simulink model "tether_model_2"  (R2021b)
settings: Solver=VariableStepAuto  StartTime=0.0  StopTime=1.5*3600  RelTol=1e-3
model workspace (MAT data in the model file):
  At = 7.85398163397e-07
  Is = 1800595238.1
  L = 5000
  a = 7378
  ecc = 0.001
  gamma = 0.00015
  h_G = 1785.71428571
  m = 350
  me = 9.1093837e-31
  mu_m = 8.22e+22
  p = 0.0031
libraries: neural x139
(part 7 of 7)

== system tether_model_2/Feed-Forward Neural Network/Layer 5/Delays 1 ==
  "p{5}" : Inport  PortDimensions=32
      mask Display: e = 0.06;c1 = [120 230 180]/255;c2 = ([120 230 180]+0)/(256+128);c3 = ([120 230 180]+128)/(256+128);patch([0 1 1 0],[0 0 1 1],c1);patch([0 1 1 1-e 1-e 0+e],[0 0 1 1-e 0+e 0+e],c2);patch([0 0 1 1-e 0+e 0+e],[0 1 1 1-e 1-e 0+e],c3);plot([0 1 1 0 0],[0 0 1 1 0]);
  mux : Mux  Inputs=1
      mask Display: e = 0.06;c1 = [120 150 230]/255;c2 = ([120 150 230]+0)/383;c3 = ([120 150 230]+128)/383;patch([0 1 1 0],[0 0 1 1],c1);patch([0 1 1 1-e 1-e 0+e],[0 0 1 1-e 0+e 0+e],c2);patch([0 0 1 1-e 0+e 0+e],[0 1 1 1-e 1-e 0+e],c3);plot([0 1 1 0 0],[0 0 1 1 0]);disp('Mux')
  "pd{5,4}" : Outport
      mask Display: e = 0.06;c1 = [120 230 180]/255;c2 = ([120 230 180]+0)/(256+128);c3 = ([120 230 180]+128)/(256+128);patch([0 1 1 0],[0 0 1 1],c1);patch([0 1 1 1-e 1-e 0+e],[0 0 1 1-e 0+e 0+e],c2);patch([0 0 1 1-e 0+e 0+e],[0 1 1 1-e 1-e 0+e],c3);plot([0 1 1 0 0],[0 0 1 1 0]);
  wires:
  "p{5}"/1 -> mux/1
  mux/1 -> "pd{5,4}"/1

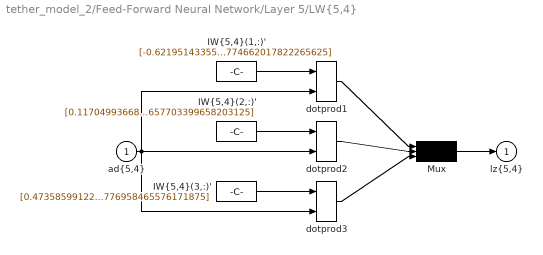
== system tether_model_2/Feed-Forward Neural Network/Layer 5/LW{5,4} ==
  "ad{5,4}" : Inport  PortDimensions=32
      mask Display: e = 0.06;c1 = [120 230 180]/255;c2 = ([120 230 180]+0)/(256+128);c3 = ([120 230 180]+128)/(256+128);patch([0 1 1 0],[0 0 1 1],c1);patch([0 1 1 1-e 1-e 0+e],[0 0 1 1-e 0+e 0+e],c2);patch([0 0 1 1-e 0+e 0+e],[0 1 1 1-e 1-e 0+e],c3);plot([0 1 1 0 0],[0 0 1 1 0]);
  "IW{5,4}(1,:)'" : Constant  Value=[-0.62195143355035809040742833531112410128116607666015625;0.204757317923436821249794093091622926294803619384765625;-0.300335195851072711548113147728145122528076171875;-0.07360812748318130982472240475544822402298450469970703125;-0.792060607860878729269415998714976012706756591796875;0.056090220190630375729501366777185467071831226348876953125;-0.460192982890725577060919704308616928756237030029296875;-0.2156401395735500770012293969557504169642925262451171875;0.3781651815348701095587102827266789972782135009765625;0.182449358825739038625357579803676344454288482666015625;-0.8124068724998851909191444065072573721408843994140625;0.99686560120035083709666423601447604596614837646484375;0.8548859964497144137141049213823862373828887939453125;0.471368357679506522206480667591677047312259674072265625;-0.74225418085054262196109675642219372093677520751953125;-0.50811740179140196804752349635236896574497222900390625;-0.08699430856769789499605138871629606001079082489013671875;0.17626293106978974112308833355200476944446563720703125;0.901505209672592844327709826757200062274932861328125;0.192819319263458577307090990871074609458446502685546875;-0.1488343844357109535536665134713985025882720947265625;-0.0743519786993882547676548711024224758148193359375;1.0321458358013513301187913384637795388698577880859375;0.1127084270811865296391118818064569495618343353271484375;-1.03056139100280663711828310624696314334869384765625;-0.81150148121102338993892999496893025934696197509765625;-0.11821508575096247029012630491706659086048603057861328125;0.08504380384017225236181758418751996941864490509033203125;0.75395417902985284452910264008096419274806976318359375;0.10092160925788225267485387348642689175903797149658203125;0.4384706426428817138685190002433955669403076171875;-0.45977774508780788753625756726250983774662017822265625]
      mask Display: e = 0.06;c1 = [120 150 230]/255;c2 = ([120 150 230]+0)/383;c3 = ([120 150 230]+128)/383;patch([0 1 1 0],[0 0 1 1],c1);patch([0 1 1 1-e 1-e 0+e],[0 0 1 1-e 0+e 0+e],c2);patch([0 0 1 1-e 0+e 0+e],[0 1 1 1-e 1-e 0+e],c3);plot([0 1 1 0 0],[0 0 1 1 0]);disp('weights');
  "IW{5,4}(2,:)'" : Constant  Value=[0.1170499366871233792863904454861767590045928955078125;-0.32708407884337187265799684610101394355297088623046875;0.478708075253142240068626733773271553218364715576171875;0.52559059568906330017767913886927999556064605712890625;0.260552228897964310849744151710183359682559967041015625;0.375021851984891851916614768924773670732975006103515625;-1.1164681773216489357736236343043856322765350341796875;0.464875249706074800126742729844409041106700897216796875;-0.360742076130005806522405009673093445599079132080078125;0.25025676258914331118177187818218953907489776611328125;0.367258700741840637959967352799139916896820068359375;-0.55567628299263327473767049013986252248287200927734375;-0.6277647777185795252563593749073334038257598876953125;-0.245924892057909294518225351566798053681850433349609375;-0.42742018018699734493992536954465322196483612060546875;0.38067959189806466202554702249472029507160186767578125;-0.2259224001307977569563689712595078162848949432373046875;-0.77198442013386381344020037431619130074977874755859375;-0.77707733974685233580004251052741892635822296142578125;0.19581128679648751589326138855540193617343902587890625;-0.45107343196972637944242023877450264990329742431640625;0.151971131808680548491707895664148963987827301025390625;0.084146090204320456162889740880928002297878265380859375;-0.1493240811492601294308002479738206602632999420166015625;-0.0304575164379494965627426239507258287630975246429443359375;-0.304097164877098091739782148579251952469348907470703125;-0.451200873198366714245111097625340335071086883544921875;0.85513455538690907875576385777094401419162750244140625;0.5945482263030330560837910525151528418064117431640625;0.48282330726073141580201308897812850773334503173828125;-0.244803318750227483224790603344445116817951202392578125;0.11076024144021918982350172200312954373657703399658203125]
      mask Display: e = 0.06;c1 = [120 150 230]/255;c2 = ([120 150 230]+0)/383;c3 = ([120 150 230]+128)/383;patch([0 1 1 0],[0 0 1 1],c1);patch([0 1 1 1-e 1-e 0+e],[0 0 1 1-e 0+e 0+e],c2);patch([0 0 1 1-e 0+e 0+e],[0 1 1 1-e 1-e 0+e],c3);plot([0 1 1 0 0],[0 0 1 1 0]);disp('weights');
  "IW{5,4}(3,:)'" : Constant  Value=[0.473585991225305813490109585472964681684970855712890625;0.6663465444866105702459435633500106632709503173828125;-0.2456992665310352708107899388778605498373508453369140625;0.378281168976102810663775244393036700785160064697265625;-0.1710741587325232127003715731916599906980991363525390625;-0.180429830712782568458152354651247151196002960205078125;-0.39599813397038918783010785773512907326221466064453125;0.289784496192740326225845137741998769342899322509765625;-0.66266444526163592598777540843002498149871826171875;0.716820604850110232320048453402705490589141845703125;-0.291571537794266755216909814407699741423130035400390625;-0.08258880437264130847108134503287146799266338348388671875;0.7348802772552149864537796020158566534519195556640625;0.729423167674049910402800378506071865558624267578125;0.50931861198151484604323968596872873604297637939453125;0.5327307495696016470532185849151574075222015380859375;0.62869955216386530505445762173621915280818939208984375;0.52236145441435455349932226454257033765316009521484375;0.9239413279772943354828385054133832454681396484375;0.394921144538807500357080471076187677681446075439453125;0.96086497796866876530685885882121510803699493408203125;0.59821828757363970652249918202869594097137451171875;0.1573707946132316681797647106577642261981964111328125;-0.219201608511633228015824670364963822066783905029296875;-0.500607302177475954607643870986066758632659912109375;0.76005796491962274163967094864347018301486968994140625;0.45021480723527229628189161303453147411346435546875;0.4763538541176599583337747390032745897769927978515625;-0.227899746591292140518447695285431109368801116943359375;0.75848112040483839368931739954859949648380279541015625;0.355304564601712835614222285585128702223300933837890625;0.4240867392359930487799601905862800776958465576171875]
      mask Display: e = 0.06;c1 = [120 150 230]/255;c2 = ([120 150 230]+0)/383;c3 = ([120 150 230]+128)/383;patch([0 1 1 0],[0 0 1 1],c1);patch([0 1 1 1-e 1-e 0+e],[0 0 1 1-e 0+e 0+e],c2);patch([0 0 1 1-e 0+e 0+e],[0 1 1 1-e 1-e 0+e],c3);plot([0 1 1 0 0],[0 0 1 1 0]);disp('weights');
  Mux : Mux  Inputs=3
      mask Display: e = 0.06;c1 = [120 150 230]/255;c2 = ([120 150 230]+0)/383;c3 = ([120 150 230]+128)/383;patch([0 1 1 0],[0 0 1 1],c1);patch([0 1 1 1-e 1-e 0+e],[0 0 1 1-e 0+e 0+e],c2);patch([0 0 1 1-e 0+e 0+e],[0 1 1 1-e 1-e 0+e],c3);plot([0 1 1 0 0],[0 0 1 1 0]);disp('Mux');
  dotprod1 : neural/Weight Functions/dotprod
  dotprod2 : neural/Weight Functions/dotprod
  dotprod3 : neural/Weight Functions/dotprod
  "lz{5,4}" : Outport
      mask Display: e = 0.06;c1 = [120 230 180]/255;c2 = ([120 230 180]+0)/(256+128);c3 = ([120 230 180]+128)/(256+128);patch([0 1 1 0],[0 0 1 1],c1);patch([0 1 1 1-e 1-e 0+e],[0 0 1 1-e 0+e 0+e],c2);patch([0 0 1 1-e 0+e 0+e],[0 1 1 1-e 1-e 0+e],c3);plot([0 1 1 0 0],[0 0 1 1 0]);
  wires:
  "IW{5,4}(1,:)'"/1 -> dotprod1/1
  "ad{5,4}"/1 -> dotprod1/2, dotprod2/2, dotprod3/2
  dotprod1/1 -> Mux/1
  "IW{5,4}(2,:)'"/1 -> dotprod2/1
  dotprod2/1 -> Mux/2
  "IW{5,4}(3,:)'"/1 -> dotprod3/1
  dotprod3/1 -> Mux/3
  Mux/1 -> "lz{5,4}"/1

== matlab function tether_model_2/MATLAB Function5 ==
  data: a input; Bx output; i input; ta input; mum input; By output; Bz output
function [Bx, By, Bz] = MagField(a, i, ta, mum)
    % Earthrs magnetic field vector in the Orbital Frame of SBET paper
    % SI units output

    % Define variables
    a = COES(1);
    i = COES(3);
    ta = COES(6);
    
%     Bo = 3.12e-5;
%     Bo_over_R3 = Bo/((p/(1+e*cos(ta)))/6378)^3;
    constant = mum/((a*1e3)^3);

    Bx = -2*constant*sin(i)*sin(ta);
    By = -constant*cos(i);
    Bz = constant*sin(i)*cos(ta);

== matlab function tether_model_2/MATLAB Function6 ==
  data: Bx input; a_r output; By input; Bz input; theta input; phi input; L input; Im input; m input; a_h output; a_theta output
function [a_r, a_h, a_theta] = edt_accelerations(Bx, By, Bz, theta, phi, L, Im, m)
    uhat = [cos(phi)*cos(theta), -sin(phi), cos(phi)*sin(theta)];
    f_orbital = Im*L*cross(uhat, [Bx, By, Bz]);
    a_orbital = f_orbital/m*1e-3'; % force to acceleraction in m to km
    a_r = a_orbital(1);
    a_h = a_orbital(2);
    a_theta = a_orbital(3);

== matlab function tether_model_2/MATLAB Function8 ==
  data: PHIe_0 input; h_0 input; Is input; ninf input; Em input; p input; At input; me input; e input; sigma input; mu input; gamma input; L input; Im output; fe output; mum input; mue_si input; h_G input
function [Im, fe] = find_current(PHIe_0, h_0, Is, ninf, Em, p, At, me, e, sigma, mu, gamma, L, mum, mue_si, h_G)
    h_span = [0, L];
    parameters = [p, At, me, Em, e, sigma, ninf, mu, gamma, h_0];
    opts = odeset( 'RelTol' , 1e-8 , 'AbsTol' , 1e-8 ) ;
    h = [];
    s = [];
    [h, s] = ode45( @current_distribution_diffe, h_span, [0, PHIe_0], opts, parameters) ;
    J1 = 0;
    Iint = 0;
    fe_right = 0;
    for ii = 2:length(h)
        J1 = J1 + ((h_G-h(ii))*(s(ii,1))+(h_G-h(ii-1))*(s(ii-1,1)))/2*(h(ii)-h(ii-1));
        Iint = Iint + (s(ii,1)+s(ii-1,1))/2*(h(ii)-h(ii-1));
        fe_right = fe_right + (h(ii)*s(ii,1) + h(ii-1)*s(ii-1,1))/2 * (h(ii)-h(ii-1));
    end
    epsilon = (J1/Is)*mum/mue_si;
    Im = Iint/L;
    fe = fe_right/(L^2*Im);

    function dstate = current_distribution_diffe(h,state,parameters) 
        Ie = real(state(1));
        PHIe = real(state(2));
    
        p = parameters(1); %perimeter in meters
        At = parameters(2);
        me = parameters(3); % mass of electron
        Em = parameters(4); % Induced electric field; dot(cross(v, B), u)
        e = parameters(5); % electron charge
        sigma = parameters(6); % from paper
        ninf = parameters(7); % ionospheric plasma density 
        mu = parameters(8); % apparently for atomic oxygen
        gamma = parameters(9);
        h0 = parameters(10);
    
        dstate = zeros(2,1);
        if real(h) < h0
            dstate(1) = e*ninf*p/pi*sqrt((2*e/me)*abs(PHIe));
        else
            dstate(1) = -e*ninf*p/pi*sqrt((2*e/me)*abs(PHIe))*mu*(1+gamma*abs(PHIe));
        end
        dstate(2) = Ie/(sigma*At)-Em;
    end
end

== matlab function tether_model_2/MATLAB Function9 ==
  data: output input; h_0 output; PHIe_0 output
function [h_0, PHIe_0] = fcn(output)

h_0 = output(1)*1e3;
PHIe_0 = output(3)*1e5;

== matlab function tether_model_2/MATLAB Function1 ==
  data: dtheta output; dphi output; Ttheta input; ddtheta output; Tphi input; Is input; theta input; phi input; dtheta input; dphi input; ddphi output
function [dtheta, dphi, ddtheta, ddphi] = fcn(Ttheta, Tphi, Is, theta, phi, dtheta, dphi)
    ddtheta = T(2)/Is;
    ddphi = T(3)/Is;

== matlab function tether_model_2/MATLAB Function ==
  data: mue input; a_r input; da output; a_h input; a_theta input; a input; ecc input; i input; RAAN input; aop input; ta input; decc output; di output; dRAAN output; daop output; dta output
function [da, decc, di, dRAAN, daop, dta]  = VoP(mue, a_r, a_h, a_theta, a, ecc, i, RAAN, aop, ta)
%     a = state(1);
%     ecc = state(2);
%     i = state(3);
%     RAAN = state(4);
%     aop = state(5);
%     ta = state(6);

    p = a*(1-ecc^2);
    h = sqrt(mue*p);
    r = p/(1+ecc*cos(ta));
    n = sqrt(mue/a^3);
    u = aop + ta;

    da = (2/(n*sqrt(1-ecc^2)))*(ecc*sin(ta)*a_r + (p/r)*a_theta);
    decc = (sqrt(1-ecc^2)/(n*a))*(sin(ta)*a_r + ...
        (cos(ta)+(ecc+cos(ta))/(1+ecc*cos(ta)))*a_theta);
    di = (r*cos(u)/(n*a^2*sqrt(1-ecc^2)))*a_h;
    dRAAN = (r*sin(u)/(n*a^2*sqrt(1-ecc^2)*sin(i)))*a_h;
    daop = (sqrt(1-ecc^2)/(n*a*ecc))*(-cos(ta)*a_r + ...
        sin(ta)*(1+r/p)*a_theta) - (r*cot(i)*sin(u)/h)*a_r;
    dta = h/r^2 + (1/(ecc*h))*(p*cos(ta)*a_r - (p+r)*sin(ta)*a_theta);

== matlab function tether_model_2/MATLAB Function2 ==
  data: theta input; Qtheta output; phi input; L input; fe input; Im input; Bx input; By input; Bz input; Qphi output
function [Qtheta, Qphi] = edt_torque(theta, phi, L, fe, Im, Bx, By, Bz)
    % x is towards zenith
    % y is -h, rotation is in-plane or theta
    % z is along track, rotation is out-of-plane or phi

    Qtheta = fe*Im*L^2*cos(phi)*(sin(phi)*(Bx*cos(theta)+Bz*sin(theta))+By*cos(phi));
    Qphi = -fe*Im*L^2*(Bx*sin(theta)-Bz*cos(theta));

== matlab function tether_model_2/MATLAB Function3 ==
  data: r input; Gtheta output; theta input; phi input; Is input; mu input; Gphi output
function [Gtheta, Gphi] = gravity_grad_torque(r, theta, phi, Is, mu)
    % Finds the gravity gradient torque effecting the tether
    % x is towards zenith
    % y is -h, rotation is in-plane or theta
    % z is along track, rotation is out-of-plane or phi
    inertia = [0, 0, 0; 0, Is, 0; 0, 0, Is];

    % Dynamics from "Spacecraft Dynamics and Control"
    u1 = [cos(phi)*cos(theta); -sin(phi); cos(phi)*sin(theta)];
    u2 = [-sin(theta); 0; cos(theta)];
    u3 = [-sin(phi)*cos(theta); -cos(phi); -sin(phi)*sin(theta)];
    tether_rotation = [u1, u2, u3];
    rb = tether_rotation*[r;0;0];

    % transform inertia into eci
    rbcross = [0, -rb(3), rb(2);
                rb(3), 0, -rb(1);
                -rb(2), rb(2), 0];
    Tgg = ((3*mu/r^5 * rbcross*inertia*rb));
    Gtheta = Tgg(2);
    Gphi = Tgg(3);

== matlab function tether_model_2/MATLAB Function4 ==
  data: a input; r output; ecc input; ta input
function r = distance_from_Earth(a, ecc, ta)
    p = a*(1-ecc^2);
    r = p/(1+ecc*cos(ta));
